simulink model "AM_SSB_SC"  (R2024a)
settings: Solver=VariableStepAuto  StartTime=0.0  StopTime=10.0  RelTol=1e-3
settings Model: Creator=zeyad  LastModifiedBy=zeyad

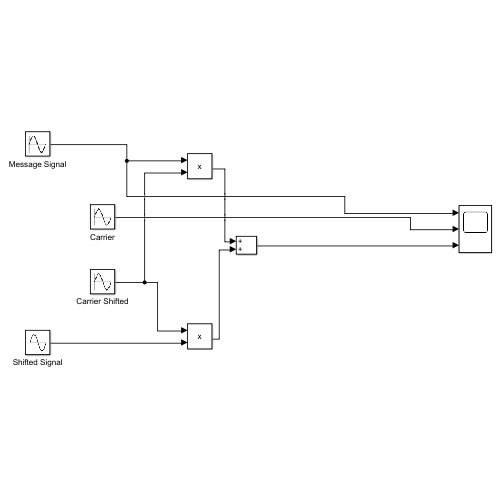
[thumbnail: Simulink's stored preview of the top-level diagram]
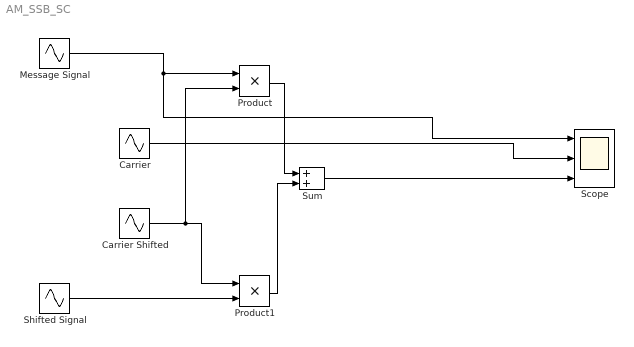
== system AM_SSB_SC ==
  Carrier : Sin  Frequency=100  SampleTime=0
  Carrier Shifted : Sin  Frequency=100  Phase=-(pi/2)  SampleTime=0
  Message Signal : Sin  Frequency=5  SampleTime=0
  Product : Product
  Product1 : Product
  Scope : Scope  NumInputPorts=3
  Shifted Signal : Sin  Frequency=5  Phase=-(pi/2)  SampleTime=0
  Sum : Sum
  wires:
  Product/1 -> Sum/1
  Product1/1 -> Sum/2
  Message Signal/1 -> Scope/1, Product/1
  Shifted Signal/1 -> Product1/2
  Carrier Shifted/1 -> Product/2, Product1/1
  Sum/1 -> Scope/3
  Carrier/1 -> Scope/2
